simulink model "Simulink_Projeto"  (R2024a)
settings: Solver=VariableStepAuto  StartTime=0.0  StopTime=6000  RelTol=1e-3
libraries: cstblocks x7
settings Model: Creator=cmcia  LastModifiedBy=cmcia

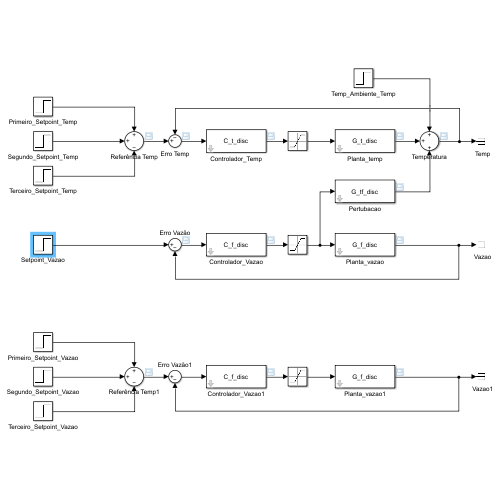
[thumbnail: Simulink's stored preview of the top-level diagram]
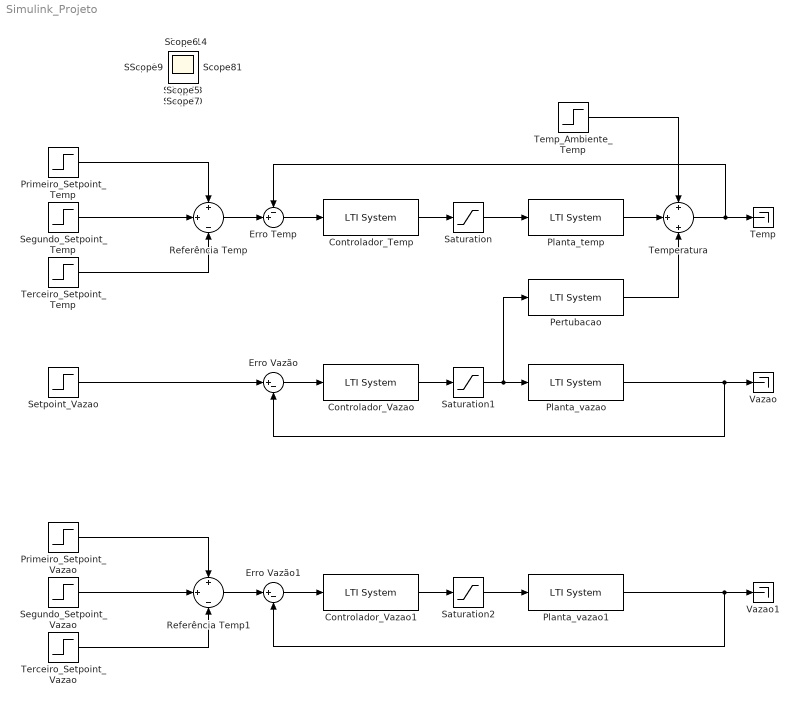
== system Simulink_Projeto ==
  Controlador_Temp : cstblocks/LTI System  sys=C_t_disc  IC=[]  PadeOrder=0
  Controlador_Vazao : cstblocks/LTI System  sys=C_f_disc  IC=[]  PadeOrder=0
  Controlador_Vazao1 : cstblocks/LTI System  sys=C_f_disc  IC=[]  PadeOrder=0
  Erro Temp : Sum  Inputs=-+|
  Erro Vazão : Sum  Inputs=|+-
  Erro Vazão1 : Sum  Inputs=|+-
  Pertubacao : cstblocks/LTI System  sys=G_tf_disc  IC=[]  PadeOrder=0
  Planta_temp : cstblocks/LTI System  sys=G_t_disc  IC=[]  PadeOrder=0
  Planta_vazao : cstblocks/LTI System  sys=G_f_disc  IC=[]  PadeOrder=0
  Planta_vazao1 : cstblocks/LTI System  sys=G_f_disc  IC=[]  PadeOrder=0
  Primeiro_Setpoint_Temp : Step  After=40  SampleTime=0
  Primeiro_Setpoint_Vazao : Step  After=20  SampleTime=0
  Referência Temp : Sum  Inputs=+|+|-
  Referência Temp1 : Sum  Inputs=+|+|-
  Saturation : Saturate  UpperLimit=255  LowerLimit=0
  Saturation1 : Saturate  UpperLimit=255  LowerLimit=0
  Saturation2 : Saturate  UpperLimit=255  LowerLimit=0
  Segundo_Setpoint_Temp : Step  Time=1900  After=5  SampleTime=0
  Segundo_Setpoint_Vazao : Step  Time=20  After=10  SampleTime=0
  Setpoint_Vazao : Step  Time=4000  After=20  SampleTime=0
  Temp : Terminator
  Temp_Ambiente_Temp : Step  After=28.12  SampleTime=0
  Temperatura : Sum  Inputs=+|+|+
  Terceiro_Setpoint_Temp : Step  Time=4000  After=10  SampleTime=0
  Terceiro_Setpoint_Vazao : Step  Time=50  After=15  SampleTime=0
  Vazao : Terminator
  Vazao1 : Terminator
  Scope{,1..14} (15 alike) : Scope
  wires:
  Controlador_Temp/1 -> Saturation/1
  Planta_vazao/1 -> Erro Vazão/2, Vazao/1
  Temperatura/1 -> Erro Temp/1, Temp/1
  Referência Temp/1 -> Erro Temp/2
  Erro Temp/1 -> Controlador_Temp/1
  Erro Vazão/1 -> Controlador_Vazao/1
  Controlador_Vazao/1 -> Saturation1/1
  Terceiro_Setpoint_Temp/1 -> Referência Temp/3
  Planta_temp/1 -> Temperatura/2
  Segundo_Setpoint_Temp/1 -> Referência Temp/2
  Primeiro_Setpoint_Temp/1 -> Referência Temp/1
  Temp_Ambiente_Temp/1 -> Temperatura/1
  Saturation/1 -> Planta_temp/1
  Pertubacao/1 -> Temperatura/3
  Setpoint_Vazao/1 -> Erro Vazão/1
  Saturation1/1 -> Pertubacao/1, Planta_vazao/1
  Controlador_Vazao1/1 -> Saturation2/1
  Saturation2/1 -> Planta_vazao1/1
  Planta_vazao1/1 -> Erro Vazão1/2, Vazao1/1
  Erro Vazão1/1 -> Controlador_Vazao1/1
  Primeiro_Setpoint_Vazao/1 -> Referência Temp1/1
  Terceiro_Setpoint_Vazao/1 -> Referência Temp1/3
  Segundo_Setpoint_Vazao/1 -> Referência Temp1/2
  Referência Temp1/1 -> Erro Vazão1/1
